simulink model "batman"  (R2024b)
settings: Solver=VariableStepAuto  StartTime=0.0  StopTime=10.0  RelTol=1e-3
libraries: sm_lib x2, nesl_utility x1
settings Model: DataDictionary=batman_dictionary.sldd  Creator=ggandolfi  LastModifiedBy=ggandolfi

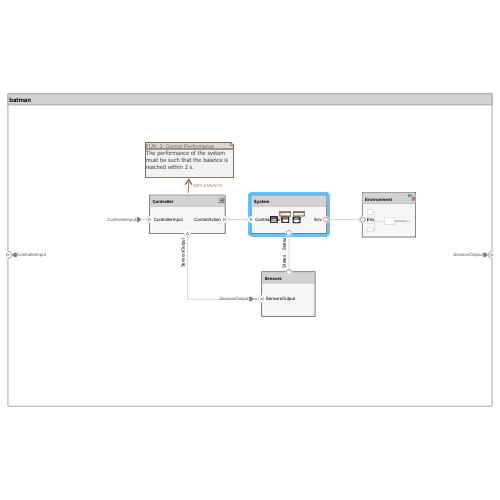
[thumbnail: Simulink's stored preview of the top-level diagram]
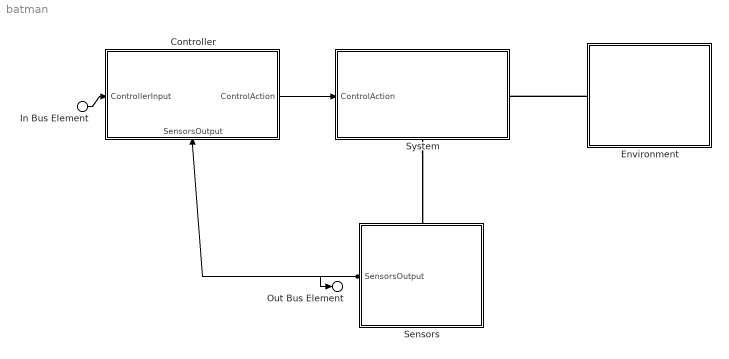
== system batman ==
  In Bus Element : Inport  PortName=ControllerInput
  Controller : Subsystem
      settings: PortSchema="{\"entries\":[{\"content\":{\"headerSize\":26,\"margin\":15,\"minimumSpacing\":25,\"sides\":[{\"content\":{\"connectorIds\":[\"In1\"]},\"type\":\"ConnectorPlacement.EquallySpacedRectSide\",\"uuid\":\"da769da6-f5f5-4696-ab2a-cae3b73f2181\"},{\"content\":{\"connectorIds\":[\"Out1\"],\"side\":\"RIGHT\"},\"type\":\"ConnectorPlacement.EquallySpacedRectSide\",\"uuid\":\"9c0a89b2-ceb4-4abb-b455-4e4ef3804a78\"},{\"content\":{\"side\":\"TOP\"},\"type\":\"ConnectorPlacement.EquallySpacedRectSide\",\"uuid\":\"9a5a1aad-ce5d-4b4f-abc9-fe7d145b0d48\"},{\"content\":{\"connectorIds\":[\"In2\"],\"side\":\"BOTTOM\"},\"type\":\"ConnectorPlacement.EquallySpacedRectSide\",\"uuid\":\"1e547295-d697-4369-8157-85ade2b38595\"}]},\"type\":\"ConnectorPlacement.EquallySpacedConnector\",\"uuid\":\"a09758ab-647a-489f-900f-f6afdfcc940e\"}],\"packageUris\":[\"http://schema.mathworks.com/mf0/Connector/R2020b\"],\"version\":\"1.0\"}"
  Environment : Subsystem
      settings: PortSchema="{\"entries\":[{\"content\":{\"headerSize\":26,\"margin\":15,\"minimumSpacing\":25,\"sides\":[{\"content\":{\"connectorIds\":[\"LConn1\"]},\"type\":\"ConnectorPlacement.EquallySpacedRectSide\",\"uuid\":\"da769da6-f5f5-4696-ab2a-cae3b73f2181\"},{\"content\":{\"side\":\"RIGHT\"},\"type\":\"ConnectorPlacement.EquallySpacedRectSide\",\"uuid\":\"9c0a89b2-ceb4-4abb-b455-4e4ef3804a78\"},{\"content\":{\"side\":\"TOP\"},\"type\":\"ConnectorPlacement.EquallySpacedRectSide\",\"uuid\":\"9a5a1aad-ce5d-4b4f-abc9-fe7d145b0d48\"}]},\"type\":\"ConnectorPlacement.EquallySpacedConnector\",\"uuid\":\"a09758ab-647a-489f-900f-f6afdfcc940e\"}],\"packageUris\":[\"http://schema.mathworks.com/mf0/Connector/R2020b\"],\"version\":\"1.0\"}"
  Sensors : Subsystem
      settings: PortSchema="{\"entries\":[{\"content\":{\"headerSize\":26,\"margin\":15,\"minimumSpacing\":25,\"sides\":[{\"content\":{\"connectorIds\":[\"Out1\"]},\"type\":\"ConnectorPlacement.EquallySpacedRectSide\",\"uuid\":\"da769da6-f5f5-4696-ab2a-cae3b73f2181\"},{\"content\":{\"side\":\"RIGHT\"},\"type\":\"ConnectorPlacement.EquallySpacedRectSide\",\"uuid\":\"9c0a89b2-ceb4-4abb-b455-4e4ef3804a78\"},{\"content\":{\"connectorIds\":[\"LConn1\"],\"side\":\"TOP\"},\"type\":\"ConnectorPlacement.EquallySpacedRectSide\",\"uuid\":\"9a5a1aad-ce5d-4b4f-abc9-fe7d145b0d48\"},{\"content\":{\"side\":\"BOTTOM\"},\"type\":\"ConnectorPlacement.EquallySpacedRectSide\",\"uuid\":\"ea03eca6-9649-4739-ba6a-01be4eb75a74\"}]},\"type\":\"ConnectorPlacement.EquallySpacedConnector\",\"uuid\":\"a09758ab-647a-489f-900f-f6afdfcc940e\"}],\"packageUris\":[\"http://schema.mathworks.com/mf0/Connector/R2020b\"],\"version\":\"1.0\"}"
  System : Subsystem
      settings: PortSchema="{\"entries\":[{\"content\":{\"headerSize\":26,\"margin\":15,\"minimumSpacing\":25,\"sides\":[{\"content\":{\"connectorIds\":[\"In1\"]},\"type\":\"ConnectorPlacement.EquallySpacedRectSide\",\"uuid\":\"da769da6-f5f5-4696-ab2a-cae3b73f2181\"},{\"content\":{\"connectorIds\":[\"RConn1\"],\"side\":\"RIGHT\"},\"type\":\"ConnectorPlacement.EquallySpacedRectSide\",\"uuid\":\"9c0a89b2-ceb4-4abb-b455-4e4ef3804a78\"},{\"content\":{\"side\":\"TOP\"},\"type\":\"ConnectorPlacement.EquallySpacedRectSide\",\"uuid\":\"9a5a1aad-ce5d-4b4f-abc9-fe7d145b0d48\"},{\"content\":{\"connectorIds\":[\"LConn1\"],\"side\":\"BOTTOM\"},\"type\":\"ConnectorPlacement.EquallySpacedRectSide\",\"uuid\":\"6d5a3914-a6f5-49fd-9ad3-8c9346453fe1\"}]},\"type\":\"ConnectorPlacement.EquallySpacedConnector\",\"uuid\":\"a09758ab-647a-489f-900f-f6afdfcc940e\"}],\"packageUris\":[\"http://schema.mathworks.com/mf0/Connector/R2020b\"],\"version\":\"1.0\"}"
  Out Bus Element : Outport  PortName=SensorsOutput
  wires:
  Controller/1(ControlAction) -> System/1(ControlAction)
  Sensors/1(SensorsOutput) -> Out Bus Element/1, Controller/2(SensorsOutput)
  In Bus Element/1 -> Controller/1(ControllerInput)
  connections:
  System/LConn1 -- Sensors/LConn1
  Environment/LConn1 -- System/RConn1

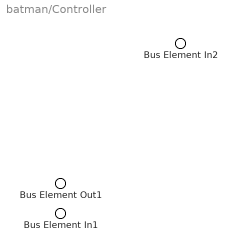
== system batman/Controller ==
  Bus Element In2 : Inport  PortName=ControllerInput
  Bus Element In1 : Inport  Port=2  PortName=SensorsOutput
  Bus Element Out1 : Outport  PortName=ControlAction

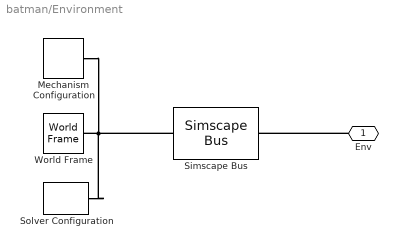
== system batman/Environment ==
  Mechanism Configuration : sm_lib/Utilities/Mechanism Configuration  UniformGravity=Constant  GravityVector=[0 0 -9.80665]  GravityVectorUnits=m/s^2  LinearizationDelta=0.001  JointModeTransitionNonlinearIterations=2
  Simscape Bus : SimscapeBus  HierarchyStrings=World  ConnectionType=Bus: Physical_Environment
  Solver Configuration : nesl_utility/Solver Configuration  PhysicalDomain=network_engine_domain  SubClassName=solver  LeftPortType=input  RightPortType=generic  Tones=[]  Harmonics=[]  SimulateNoise=off  Profile=off  UseLocalSampling=off  EnableSwitchedLinearOptims=on  FrequencyDomain=off  UseCCode=off  RelTol=0.001  AbsTol=0.001  MinStep=1e-09  ToWorkspace=off  RevertToSquareIcSolve=off  NumHomotopyIterations=100  PhasorMode=off  PhasorModeNumHarmonics=1  ConsistencySolver=NEWTON_XTOL_AFTER_FTOL  IndexReductionMethod=DerivativeReplacement  DoDC=off  ResidualTolerance=1e-09  ConsistencyTolSource=GLOBAL  ConsistencyAbsTol=0.001  ConsistencyRelTol=0.001  ConsistencyTolFactor=0.001  UseLocalSolver=off  LocalSolverChoice=NE_BACKWARD_EULER_ADVANCER  ResolveIndetEquations=on  FunctionEvalNumThread=1  LocalSolverSampleTime=0.001  DoFixedCost=off  MaxNonlinIter=3  MaxModeIter=2  ComputeImpulses=off  ImpulseIterations=2  LinearAlgebra=auto  LinearAlgebraNumThread=0  EquationFormulation=NE_TIME_EF  DelaysMemoryBudget=1024  AutomaticFiltering=on  FilteringTimeConstant=0.001  PartitionStorageMethod=AS_NEEDED  PartitionMemoryBudget=1024  PartitionMethod=ROBUST  MultibodyUseLocalSolver=off  MultibodyLocalSolverChoice=ODE1  MultibodyLocalSolverSampleTime=0.001
  World Frame : sm_lib/Frames and Transforms/World Frame
  Env : PMIOPort  Side=Left  ConnectionType=Bus: Physical_Environment
  connections:
  Mechanism Configuration/RConn1 -- Simscape Bus/LConn1 -- Solver Configuration/RConn1 -- World Frame/RConn1
  Env/RConn1 -- Simscape Bus/RConn1

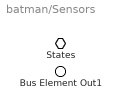
== system batman/Sensors ==
  States : PMIOPort  Side=Left  ConnectionType=Bus: Physical_SystemStates
  Bus Element Out1 : Outport  PortName=SensorsOutput

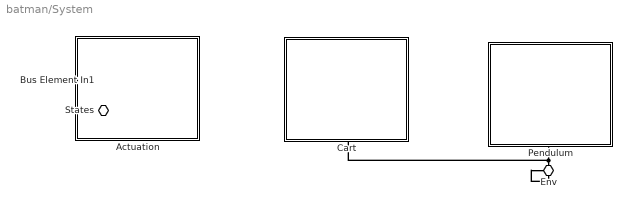
== system batman/System ==
  Bus Element In1 : Inport  PortName=ControlAction
  Actuation : Subsystem
      settings: PortSchema="{\"entries\":[{\"content\":{\"headerSize\":26,\"margin\":15,\"minimumSpacing\":25,\"sides\":[{\"content\":{},\"type\":\"ConnectorPlacement.EquallySpacedRectSide\",\"uuid\":\"da769da6-f5f5-4696-ab2a-cae3b73f2181\"},{\"content\":{\"side\":\"RIGHT\"},\"type\":\"ConnectorPlacement.EquallySpacedRectSide\",\"uuid\":\"9c0a89b2-ceb4-4abb-b455-4e4ef3804a78\"},{\"content\":{\"side\":\"TOP\"},\"type\":\"ConnectorPlacement.EquallySpacedRectSide\",\"uuid\":\"9a5a1aad-ce5d-4b4f-abc9-fe7d145b0d48\"}]},\"type\":\"ConnectorPlacement.EquallySpacedConnector\",\"uuid\":\"a09758ab-647a-489f-900f-f6afdfcc940e\"}],\"packageUris\":[\"http://schema.mathworks.com/mf0/Connector/R2020b\"],\"version\":\"1.0\"}"
  Cart : Subsystem  ReferencedSubsystem=Cart
      settings: PortSchema="{\"entries\":[{\"content\":{\"headerSize\":26,\"margin\":15,\"minimumSpacing\":25,\"sides\":[{\"content\":{},\"type\":\"ConnectorPlacement.EquallySpacedRectSide\",\"uuid\":\"da769da6-f5f5-4696-ab2a-cae3b73f2181\"},{\"content\":{\"side\":\"RIGHT\"},\"type\":\"ConnectorPlacement.EquallySpacedRectSide\",\"uuid\":\"9c0a89b2-ceb4-4abb-b455-4e4ef3804a78\"},{\"content\":{\"side\":\"TOP\"},\"type\":\"ConnectorPlacement.EquallySpacedRectSide\",\"uuid\":\"9a5a1aad-ce5d-4b4f-abc9-fe7d145b0d48\"},{\"content\":{\"connectorIds\":[\"RConn1\"],\"side\":\"BOTTOM\"},\"type\":\"ConnectorPlacement.EquallySpacedRectSide\",\"uuid\":\"e5edd7e2-ee06-4c35-88b3-febbe34a8028\"}]},\"type\":\"ConnectorPlacement.EquallySpacedConnector\",\"uuid\":\"a09758ab-647a-489f-900f-f6afdfcc940e\"}],\"packageUris\":[\"http://schema.mathworks.com/mf0/Connector/R2020b\"],\"version\":\"1.0\"}"
  Pendulum : Subsystem  ReferencedSubsystem=Pendulum
      settings: PortSchema="{\"entries\":[{\"content\":{\"headerSize\":26,\"margin\":15,\"minimumSpacing\":25,\"sides\":[{\"content\":{},\"type\":\"ConnectorPlacement.EquallySpacedRectSide\",\"uuid\":\"da769da6-f5f5-4696-ab2a-cae3b73f2181\"},{\"content\":{\"side\":\"RIGHT\"},\"type\":\"ConnectorPlacement.EquallySpacedRectSide\",\"uuid\":\"9c0a89b2-ceb4-4abb-b455-4e4ef3804a78\"},{\"content\":{\"side\":\"TOP\"},\"type\":\"ConnectorPlacement.EquallySpacedRectSide\",\"uuid\":\"9a5a1aad-ce5d-4b4f-abc9-fe7d145b0d48\"},{\"content\":{\"connectorIds\":[\"RConn1\"],\"side\":\"BOTTOM\"},\"type\":\"ConnectorPlacement.EquallySpacedRectSide\",\"uuid\":\"0549c167-9738-45da-8272-fe4c1623cae2\"}]},\"type\":\"ConnectorPlacement.EquallySpacedConnector\",\"uuid\":\"a09758ab-647a-489f-900f-f6afdfcc940e\"}],\"packageUris\":[\"http://schema.mathworks.com/mf0/Connector/R2020b\"],\"version\":\"1.0\"}"
  States : PMIOPort  Side=Left  ConnectionType=Bus: Physical_SystemStates
  Env : PMIOPort  Port=2  Side=Right  ConnectionType=Bus: Physical_Environment
  connections:
  Env/RConn1 -- Pendulum/RConn1 -- Cart/RConn1

== system batman/System/Actuation ==
